simulink model "Fusion_Frame_Model_Architecture"  (R2018a)
settings: Solver=FixedStepAuto  StartTime=0.0  StopTime=SimulationTime  FixedStep=SamplingTime  RelTol=1e-3
undefined symbols (not defined in the file or in its folder): ACTIVATE_CAM, ACTIVATE_RAD, CAM1_detTimeStamp, CAM1_MeasNoise, CAM1_objClassID, CAM1_PX, CAM1_PY, CAM1_VX, CAM1_VY, CAM2_detTimeStamp, CAM2_MeasNoise, CAM2_objClassID, CAM2_PX, CAM2_PY, CAM2_VX, CAM2_VY, CAM3_detTimeStamp, CAM3_MeasNoise, CAM3_objClassID, CAM3_PX, CAM3_PY, CAM3_VX, CAM3_VY, CAM4_detTimeStamp, CAM4_MeasNoise, CAM4_objClassID, CAM4_PX, CAM4_PY, CAM4_VX, CAM4_VY, CAM5_detTimeStamp, CAM5_MeasNoise, CAM5_objClassID, CAM5_PX, CAM5_PY, CAM5_VX, CAM5_VY, CAM6_detTimeStamp, CAM6_MeasNoise, CAM6_objClassID, CAM6_PX, CAM6_PY, CAM6_VX, CAM6_VY, CAM7_detTimeStamp, CAM7_MeasNoise, CAM7_objClassID, CAM7_PX, CAM7_PY, CAM7_VX, CAM7_VY, CAM8_detTimeStamp, CAM8_MeasNoise, CAM8_objClassID, CAM8_PX, CAM8_PY, CAM8_VX, CAM8_VY, CAM_nMeas, CAM_TYPE ... (+181)
libraries: simulink_extras x4
(part 7 of 11)

== system Fusion_Frame_Model_Architecture/SENSOR_MEASUREMENTS/RADAR_CAMERA_EGO_SENSOR_INTERFACE/RoadSensors/Camera6/ExtractMeasParam1 ==
  idx : Inport
  time : Inport  Port=2
  Constant : Constant  Value=LINE_CURVATURE_CAM6
  Constant1 : Constant  Value=LINE_CURVDERIVATIVE_CAM6
  Constant2 : Constant  Value=LINE_CURVELENGTH_CAM6
  Constant3 : Constant  Value=LINE_HEADINGANGLE_CAM6
  Constant4 : Constant  Value=LINE_LATERALOFFSET_CAM6
  Constant5 : Constant  Value=LINE_XMIN_CAM6
  Constant6 : Constant  Value=LINE_detTimeStamp_CAM6
  Constant7 : Constant  Value=LINE_XMAX_CAM6
  Constant8 : Constant  Value=LINE_WIDTH_CAM6
  CurvLength : Selector  NumberOfDimensions=2  InputPortWidth=3  IndexOptions=Index vector (port),Index vector (port)  Indices=[1 3],1  OutputSizes=1,1
  Curvature : Selector  NumberOfDimensions=2  InputPortWidth=3  IndexOptions=Index vector (port),Index vector (port)  Indices=[1 3],1  OutputSizes=1,1
  CurvatureRate : Selector  NumberOfDimensions=2  InputPortWidth=3  IndexOptions=Index vector (port),Index vector (port)  Indices=[1 3],1  OutputSizes=1,1
  HeadingAngle : Selector  NumberOfDimensions=2  InputPortWidth=3  IndexOptions=Index vector (port),Index vector (port)  Indices=[1 3],1  OutputSizes=1,1
  LateralOffset : Selector  NumberOfDimensions=2  InputPortWidth=3  IndexOptions=Index vector (port),Index vector (port)  Indices=[1 3],1  OutputSizes=1,1
  lineWidth : Selector  NumberOfDimensions=2  InputPortWidth=3  IndexOptions=Index vector (port),Index vector (port)  Indices=[1 3],1  OutputSizes=1,1
  minValidX : Selector  NumberOfDimensions=2  InputPortWidth=3  IndexOptions=Index vector (port),Index vector (port)  Indices=[1 3],1  OutputSizes=1,1
  minValidY : Selector  NumberOfDimensions=2  InputPortWidth=3  IndexOptions=Index vector (port),Index vector (port)  Indices=[1 3],1  OutputSizes=1,1
  timeStamp : Selector  NumberOfDimensions=2  InputPortWidth=3  IndexOptions=Select all,Index vector (port)  Indices=[1 3],1  OutputSizes=1,1
  curvature : Outport
  curvRate : Outport  Port=2
  curvLength : Outport  Port=3
  headingAngle : Outport  Port=4
  lateralOffset : Outport  Port=5
  xmin : Outport  Port=6
  xmax : Outport  Port=7
  lineMarkWidth : Outport  Port=8
  measCaptureTime : Outport  Port=9
  wires:
  Constant3/1 -> HeadingAngle/1
  Constant2/1 -> CurvLength/1
  HeadingAngle/1 -> headingAngle/1
  Constant/1 -> Curvature/1
  Constant1/1 -> CurvatureRate/1
  CurvLength/1 -> curvLength/1
  Curvature/1 -> curvature/1
  CurvatureRate/1 -> curvRate/1
  Constant4/1 -> LateralOffset/1
  Constant5/1 -> minValidX/1
  Constant6/1 -> timeStamp/1
  timeStamp/1 -> measCaptureTime/1
  minValidX/1 -> xmin/1
  LateralOffset/1 -> lateralOffset/1
  minValidY/1 -> xmax/1
  Constant7/1 -> minValidY/1
  lineWidth/1 -> lineMarkWidth/1
  time/1 -> minValidX/2, minValidY/2, lineWidth/2, timeStamp/2, LateralOffset/2, HeadingAngle/2, CurvLength/2, CurvatureRate/2, Curvature/2
  idx/1 -> minValidX/3, lineWidth/3, minValidY/3, LateralOffset/3, HeadingAngle/3, CurvLength/3, CurvatureRate/3, Curvature/3
  Constant8/1 -> lineWidth/1

== system Fusion_Frame_Model_Architecture/SENSOR_MEASUREMENTS/RADAR_CAMERA_EGO_SENSOR_INTERFACE/RoadSensors/Camera6/IsValid2 ==
  LineID : Inport
  curvature : Inport  Port=2
  curvatureRate : Inport  Port=3
  curvLength : Inport  Port=4
  HeadingAngle : Inport  Port=5
  Abs{,1..3} (4 alike) : Abs
  Add : Sum  Inputs=++++
  Constant : Constant  Value=uint16(0)
  Data Type Conversion : DataTypeConversion  OutDataTypeStr=uint16
  Switch : Switch  Threshold=0.000001
  validID : Outport
  wires:
  Add/1 -> Switch/2
  Abs2/1 -> Add/3
  Constant/1 -> Switch/3
  Abs/1 -> Add/1
  curvature/1 -> Abs/1
  Abs3/1 -> Add/4
  Abs1/1 -> Add/2
  HeadingAngle/1 -> Abs3/1
  curvatureRate/1 -> Abs1/1
  curvLength/1 -> Abs2/1
  LineID/1 -> Data Type Conversion/1
  Switch/1 -> validID/1
  Data Type Conversion/1 -> Switch/1

== system Fusion_Frame_Model_Architecture/SENSOR_MEASUREMENTS/RADAR_CAMERA_EGO_SENSOR_INTERFACE/RoadSensors/Camera6/Subsystem1 ==
  CameraLineCoeff : Inport
  curv : Inport  Port=2
  curvRate : Inport  Port=3
  curvLen : Inport  Port=4
  alpha : Inport  Port=5
  ValidID : Inport  Port=6
  lateralOffset : Inport  Port=7
  xmin : Inport  Port=8
  xmax : Inport  Port=9
  lineWidth : Inport  Port=10
  TIME_STAMP : Inport  Port=11
  iter : Inport  Port=12
  Assignment : Assignment  DiagnosticForDimensions=Warning  IndexOptions=Index vector (port)  Indices=1  OutputSizes=1
  Bus Creator1 : BusCreator  Inputs=11  OutDataTypeStr=Bus: LineMeasParam  NonVirtualBus=on
  Bus Creator2 : BusCreator  Inputs=11  OutDataTypeStr=Bus: LineMeasParam  NonVirtualBus=on
  Constant1 : Constant  Value=single(10)
  Constant14 : Constant  Value=uint8(6)
  Constant2 : Constant  Value=single(10)
  Constant{35..39,43} (6 alike) : Constant  Value=single(0)
  Constant44 : Constant  Value=single(10)
  Switch : Switch  Criteria=u2 ~= 0
  C1 : Outport
  wires:
  Bus Creator1/1 -> Switch/3
  ValidID/1 -> Bus Creator1/2, Switch/2, Bus Creator2/2  "lineID"
  Bus Creator2/1 -> Switch/1
  CameraLineCoeff/1 -> Assignment/1
  Switch/1 -> Assignment/2
  iter/1 -> Assignment/3
  Assignment/1 -> C1/1
  TIME_STAMP/1 -> Bus Creator2/1  "TimeStamp"
  curv/1 -> Bus Creator2/4  "curvature"
  curvRate/1 -> Bus Creator2/5  "curvatureRate"
  curvLen/1 -> Bus Creator2/6  "curveLength"
  alpha/1 -> Bus Creator2/7  "HeadingAngle"
  lateralOffset/1 -> Bus Creator2/8  "LateralOffset"
  lineWidth/1 -> Bus Creator2/11  "LineMarkWidth"
  xmax/1 -> Bus Creator2/10  "validMinLongCoordLine"
  xmin/1 -> Bus Creator2/9  "validMaxLongCoordLine"
  Constant35/1 -> Bus Creator1/1  "TimeStamp"
  Constant14/1 -> Bus Creator2/3, Bus Creator1/3  "cameraID"
  Constant36/1 -> Bus Creator1/4  "curvature"
  Constant37/1 -> Bus Creator1/5  "curvatureRate"
  Constant38/1 -> Bus Creator1/6  "curveLength"
  Constant39/1 -> Bus Creator1/7  "HeadingAngle"
  Constant43/1 -> Bus Creator1/8  "LateralOffset"
  Constant44/1 -> Bus Creator1/9  "validMaxLongCoordLine"
  Constant1/1 -> Bus Creator1/10  "validMinLongCoordLine"
  Constant2/1 -> Bus Creator1/11  "LineMarkWidth"

== system Fusion_Frame_Model_Architecture/SENSOR_MEASUREMENTS/RADAR_CAMERA_EGO_SENSOR_INTERFACE/RoadSensors/Camera7/ExtractMeasParam1 ==
  idx : Inport
  time : Inport  Port=2
  Constant : Constant  Value=LINE_CURVATURE_CAM7
  Constant1 : Constant  Value=LINE_CURVDERIVATIVE_CAM7
  Constant2 : Constant  Value=LINE_CURVELENGTH_CAM7
  Constant3 : Constant  Value=LINE_HEADINGANGLE_CAM7
  Constant4 : Constant  Value=LINE_LATERALOFFSET_CAM7
  Constant5 : Constant  Value=LINE_XMIN_CAM7
  Constant6 : Constant  Value=LINE_detTimeStamp_CAM7
  Constant7 : Constant  Value=LINE_XMAX_CAM7
  Constant8 : Constant  Value=LINE_WIDTH_CAM7
  CurvLength : Selector  NumberOfDimensions=2  InputPortWidth=3  IndexOptions=Index vector (port),Index vector (port)  Indices=[1 3],1  OutputSizes=1,1
  Curvature : Selector  NumberOfDimensions=2  InputPortWidth=3  IndexOptions=Index vector (port),Index vector (port)  Indices=[1 3],1  OutputSizes=1,1
  CurvatureRate : Selector  NumberOfDimensions=2  InputPortWidth=3  IndexOptions=Index vector (port),Index vector (port)  Indices=[1 3],1  OutputSizes=1,1
  HeadingAngle : Selector  NumberOfDimensions=2  InputPortWidth=3  IndexOptions=Index vector (port),Index vector (port)  Indices=[1 3],1  OutputSizes=1,1
  LateralOffset : Selector  NumberOfDimensions=2  InputPortWidth=3  IndexOptions=Index vector (port),Index vector (port)  Indices=[1 3],1  OutputSizes=1,1
  lineWidth : Selector  NumberOfDimensions=2  InputPortWidth=3  IndexOptions=Index vector (port),Index vector (port)  Indices=[1 3],1  OutputSizes=1,1
  minValidX : Selector  NumberOfDimensions=2  InputPortWidth=3  IndexOptions=Index vector (port),Index vector (port)  Indices=[1 3],1  OutputSizes=1,1
  minValidY : Selector  NumberOfDimensions=2  InputPortWidth=3  IndexOptions=Index vector (port),Index vector (port)  Indices=[1 3],1  OutputSizes=1,1
  timeStamp : Selector  NumberOfDimensions=2  InputPortWidth=3  IndexOptions=Select all,Index vector (port)  Indices=[1 3],1  OutputSizes=1,1
  curvature : Outport
  curvRate : Outport  Port=2
  curvLength : Outport  Port=3
  headingAngle : Outport  Port=4
  lateralOffset : Outport  Port=5
  xmin : Outport  Port=6
  xmax : Outport  Port=7
  lineMarkWidth : Outport  Port=8
  measCaptureTime : Outport  Port=9
  wires:
  Constant3/1 -> HeadingAngle/1
  Constant2/1 -> CurvLength/1
  HeadingAngle/1 -> headingAngle/1
  Constant/1 -> Curvature/1
  Constant1/1 -> CurvatureRate/1
  CurvLength/1 -> curvLength/1
  Curvature/1 -> curvature/1
  CurvatureRate/1 -> curvRate/1
  Constant4/1 -> LateralOffset/1
  Constant5/1 -> minValidX/1
  Constant6/1 -> timeStamp/1
  timeStamp/1 -> measCaptureTime/1
  minValidX/1 -> xmin/1
  LateralOffset/1 -> lateralOffset/1
  minValidY/1 -> xmax/1
  Constant7/1 -> minValidY/1
  lineWidth/1 -> lineMarkWidth/1
  time/1 -> minValidX/2, minValidY/2, lineWidth/2, timeStamp/2, LateralOffset/2, HeadingAngle/2, CurvLength/2, CurvatureRate/2, Curvature/2
  idx/1 -> minValidX/3, lineWidth/3, minValidY/3, LateralOffset/3, HeadingAngle/3, CurvLength/3, CurvatureRate/3, Curvature/3
  Constant8/1 -> lineWidth/1

== system Fusion_Frame_Model_Architecture/SENSOR_MEASUREMENTS/RADAR_CAMERA_EGO_SENSOR_INTERFACE/RoadSensors/Camera7/IsValid2 ==
  LineID : Inport
  curvature : Inport  Port=2
  curvatureRate : Inport  Port=3
  curvLength : Inport  Port=4
  HeadingAngle : Inport  Port=5
  Abs{,1..3} (4 alike) : Abs
  Add : Sum  Inputs=++++
  Constant : Constant  Value=uint16(0)
  Data Type Conversion : DataTypeConversion  OutDataTypeStr=uint16
  Switch : Switch  Threshold=0.000001
  validID : Outport
  wires:
  Add/1 -> Switch/2
  Abs2/1 -> Add/3
  Constant/1 -> Switch/3
  Abs/1 -> Add/1
  curvature/1 -> Abs/1
  Abs3/1 -> Add/4
  Abs1/1 -> Add/2
  HeadingAngle/1 -> Abs3/1
  curvatureRate/1 -> Abs1/1
  curvLength/1 -> Abs2/1
  LineID/1 -> Data Type Conversion/1
  Switch/1 -> validID/1
  Data Type Conversion/1 -> Switch/1

== system Fusion_Frame_Model_Architecture/SENSOR_MEASUREMENTS/RADAR_CAMERA_EGO_SENSOR_INTERFACE/RoadSensors/Camera7/Subsystem1 ==
  CameraLineCoeff : Inport
  curv : Inport  Port=2
  curvRate : Inport  Port=3
  curvLen : Inport  Port=4
  alpha : Inport  Port=5
  ValidID : Inport  Port=6
  lateralOffset : Inport  Port=7
  xmin : Inport  Port=8
  xmax : Inport  Port=9
  lineWidth : Inport  Port=10
  TIME_STAMP : Inport  Port=11
  iter : Inport  Port=12
  Assignment : Assignment  DiagnosticForDimensions=Warning  IndexOptions=Index vector (port)  Indices=1  OutputSizes=1
  Bus Creator1 : BusCreator  Inputs=11  OutDataTypeStr=Bus: LineMeasParam  NonVirtualBus=on
  Bus Creator2 : BusCreator  Inputs=11  OutDataTypeStr=Bus: LineMeasParam  NonVirtualBus=on
  Constant1 : Constant  Value=single(10)
  Constant14 : Constant  Value=uint8(7)
  Constant2 : Constant  Value=single(10)
  Constant{35..39,43} (6 alike) : Constant  Value=single(0)
  Constant44 : Constant  Value=single(10)
  Switch : Switch  Criteria=u2 ~= 0
  C1 : Outport
  wires:
  Bus Creator1/1 -> Switch/3
  ValidID/1 -> Bus Creator1/2, Switch/2, Bus Creator2/2  "lineID"
  Bus Creator2/1 -> Switch/1
  CameraLineCoeff/1 -> Assignment/1
  Switch/1 -> Assignment/2
  iter/1 -> Assignment/3
  Assignment/1 -> C1/1
  TIME_STAMP/1 -> Bus Creator2/1  "TimeStamp"
  curv/1 -> Bus Creator2/4  "curvature"
  curvRate/1 -> Bus Creator2/5  "curvatureRate"
  curvLen/1 -> Bus Creator2/6  "curveLength"
  alpha/1 -> Bus Creator2/7  "HeadingAngle"
  lateralOffset/1 -> Bus Creator2/8  "LateralOffset"
  lineWidth/1 -> Bus Creator2/11  "LineMarkWidth"
  xmax/1 -> Bus Creator2/10  "validMinLongCoordLine"
  xmin/1 -> Bus Creator2/9  "validMaxLongCoordLine"
  Constant35/1 -> Bus Creator1/1  "TimeStamp"
  Constant14/1 -> Bus Creator2/3, Bus Creator1/3  "cameraID"
  Constant36/1 -> Bus Creator1/4  "curvature"
  Constant37/1 -> Bus Creator1/5  "curvatureRate"
  Constant38/1 -> Bus Creator1/6  "curveLength"
  Constant39/1 -> Bus Creator1/7  "HeadingAngle"
  Constant43/1 -> Bus Creator1/8  "LateralOffset"
  Constant44/1 -> Bus Creator1/9  "validMaxLongCoordLine"
  Constant1/1 -> Bus Creator1/10  "validMinLongCoordLine"
  Constant2/1 -> Bus Creator1/11  "LineMarkWidth"

== system Fusion_Frame_Model_Architecture/SENSOR_MEASUREMENTS/RADAR_CAMERA_EGO_SENSOR_INTERFACE/RoadSensors/Camera8/ExtractMeasParam1 ==
  idx : Inport
  time : Inport  Port=2
  Constant : Constant  Value=LINE_CURVATURE_CAM8
  Constant1 : Constant  Value=LINE_CURVDERIVATIVE_CAM8
  Constant2 : Constant  Value=LINE_CURVELENGTH_CAM8
  Constant3 : Constant  Value=LINE_HEADINGANGLE_CAM8
  Constant4 : Constant  Value=LINE_LATERALOFFSET_CAM8
  Constant5 : Constant  Value=LINE_XMIN_CAM8
  Constant6 : Constant  Value=LINE_detTimeStamp_CAM8
  Constant7 : Constant  Value=LINE_XMAX_CAM8
  Constant8 : Constant  Value=LINE_WIDTH_CAM8
  CurvLength : Selector  NumberOfDimensions=2  InputPortWidth=3  IndexOptions=Index vector (port),Index vector (port)  Indices=[1 3],1  OutputSizes=1,1
  Curvature : Selector  NumberOfDimensions=2  InputPortWidth=3  IndexOptions=Index vector (port),Index vector (port)  Indices=[1 3],1  OutputSizes=1,1
  CurvatureRate : Selector  NumberOfDimensions=2  InputPortWidth=3  IndexOptions=Index vector (port),Index vector (port)  Indices=[1 3],1  OutputSizes=1,1
  HeadingAngle : Selector  NumberOfDimensions=2  InputPortWidth=3  IndexOptions=Index vector (port),Index vector (port)  Indices=[1 3],1  OutputSizes=1,1
  LateralOffset : Selector  NumberOfDimensions=2  InputPortWidth=3  IndexOptions=Index vector (port),Index vector (port)  Indices=[1 3],1  OutputSizes=1,1
  lineWidth : Selector  NumberOfDimensions=2  InputPortWidth=3  IndexOptions=Index vector (port),Index vector (port)  Indices=[1 3],1  OutputSizes=1,1
  minValidX : Selector  NumberOfDimensions=2  InputPortWidth=3  IndexOptions=Index vector (port),Index vector (port)  Indices=[1 3],1  OutputSizes=1,1
  minValidY : Selector  NumberOfDimensions=2  InputPortWidth=3  IndexOptions=Index vector (port),Index vector (port)  Indices=[1 3],1  OutputSizes=1,1
  timeStamp : Selector  NumberOfDimensions=2  InputPortWidth=3  IndexOptions=Select all,Index vector (port)  Indices=[1 3],1  OutputSizes=1,1
  curvature : Outport
  curvRate : Outport  Port=2
  curvLength : Outport  Port=3
  headingAngle : Outport  Port=4
  lateralOffset : Outport  Port=5
  xmin : Outport  Port=6
  xmax : Outport  Port=7
  lineMarkWidth : Outport  Port=8
  measCaptureTime : Outport  Port=9
  wires:
  Constant3/1 -> HeadingAngle/1
  Constant2/1 -> CurvLength/1
  HeadingAngle/1 -> headingAngle/1
  Constant/1 -> Curvature/1
  Constant1/1 -> CurvatureRate/1
  CurvLength/1 -> curvLength/1
  Curvature/1 -> curvature/1
  CurvatureRate/1 -> curvRate/1
  Constant4/1 -> LateralOffset/1
  Constant5/1 -> minValidX/1
  Constant6/1 -> timeStamp/1
  timeStamp/1 -> measCaptureTime/1
  minValidX/1 -> xmin/1
  LateralOffset/1 -> lateralOffset/1
  minValidY/1 -> xmax/1
  Constant7/1 -> minValidY/1
  lineWidth/1 -> lineMarkWidth/1
  time/1 -> minValidX/2, minValidY/2, lineWidth/2, timeStamp/2, LateralOffset/2, HeadingAngle/2, CurvLength/2, CurvatureRate/2, Curvature/2
  idx/1 -> minValidX/3, lineWidth/3, minValidY/3, LateralOffset/3, HeadingAngle/3, CurvLength/3, CurvatureRate/3, Curvature/3
  Constant8/1 -> lineWidth/1

== system Fusion_Frame_Model_Architecture/SENSOR_MEASUREMENTS/RADAR_CAMERA_EGO_SENSOR_INTERFACE/RoadSensors/Camera8/IsValid2 ==
  LineID : Inport
  curvature : Inport  Port=2
  curvatureRate : Inport  Port=3
  curvLength : Inport  Port=4
  HeadingAngle : Inport  Port=5
  Abs{,1..3} (4 alike) : Abs
  Add : Sum  Inputs=++++
  Constant : Constant  Value=uint16(0)
  Data Type Conversion : DataTypeConversion  OutDataTypeStr=uint16
  Switch : Switch  Threshold=0.000001
  validID : Outport
  wires:
  Add/1 -> Switch/2
  Abs2/1 -> Add/3
  Constant/1 -> Switch/3
  Abs/1 -> Add/1
  curvature/1 -> Abs/1
  Abs3/1 -> Add/4
  Abs1/1 -> Add/2
  HeadingAngle/1 -> Abs3/1
  curvatureRate/1 -> Abs1/1
  curvLength/1 -> Abs2/1
  LineID/1 -> Data Type Conversion/1
  Switch/1 -> validID/1
  Data Type Conversion/1 -> Switch/1

== system Fusion_Frame_Model_Architecture/SENSOR_MEASUREMENTS/RADAR_CAMERA_EGO_SENSOR_INTERFACE/RoadSensors/Camera8/Subsystem1 ==
  CameraLineCoeff : Inport
  curv : Inport  Port=2
  curvRate : Inport  Port=3
  curvLen : Inport  Port=4
  alpha : Inport  Port=5
  ValidID : Inport  Port=6
  lateralOffset : Inport  Port=7
  xmin : Inport  Port=8
  xmax : Inport  Port=9
  lineWidth : Inport  Port=10
  TIME_STAMP : Inport  Port=11
  iter : Inport  Port=12
  Assignment : Assignment  DiagnosticForDimensions=Warning  IndexOptions=Index vector (port)  Indices=1  OutputSizes=1
  Bus Creator1 : BusCreator  Inputs=11  OutDataTypeStr=Bus: LineMeasParam  NonVirtualBus=on
  Bus Creator2 : BusCreator  Inputs=11  OutDataTypeStr=Bus: LineMeasParam  NonVirtualBus=on
  Constant1 : Constant  Value=single(10)
  Constant14 : Constant  Value=uint8(8)
  Constant2 : Constant  Value=single(10)
  Constant{35..39,43} (6 alike) : Constant  Value=single(0)
  Constant44 : Constant  Value=single(10)
  Switch : Switch  Criteria=u2 ~= 0
  C1 : Outport
  wires:
  Bus Creator1/1 -> Switch/3
  ValidID/1 -> Bus Creator1/2, Switch/2, Bus Creator2/2  "lineID"
  Bus Creator2/1 -> Switch/1
  CameraLineCoeff/1 -> Assignment/1
  Switch/1 -> Assignment/2
  iter/1 -> Assignment/3
  Assignment/1 -> C1/1
  TIME_STAMP/1 -> Bus Creator2/1  "TimeStamp"
  curv/1 -> Bus Creator2/4  "curvature"
  curvRate/1 -> Bus Creator2/5  "curvatureRate"
  curvLen/1 -> Bus Creator2/6  "curveLength"
  alpha/1 -> Bus Creator2/7  "HeadingAngle"
  lateralOffset/1 -> Bus Creator2/8  "LateralOffset"
  lineWidth/1 -> Bus Creator2/11  "LineMarkWidth"
  xmax/1 -> Bus Creator2/10  "validMinLongCoordLine"
  xmin/1 -> Bus Creator2/9  "validMaxLongCoordLine"
  Constant35/1 -> Bus Creator1/1  "TimeStamp"
  Constant14/1 -> Bus Creator2/3, Bus Creator1/3  "cameraID"
  Constant36/1 -> Bus Creator1/4  "curvature"
  Constant37/1 -> Bus Creator1/5  "curvatureRate"
  Constant38/1 -> Bus Creator1/6  "curveLength"
  Constant39/1 -> Bus Creator1/7  "HeadingAngle"
  Constant43/1 -> Bus Creator1/8  "LateralOffset"
  Constant44/1 -> Bus Creator1/9  "validMaxLongCoordLine"
  Constant1/1 -> Bus Creator1/10  "validMinLongCoordLine"
  Constant2/1 -> Bus Creator1/11  "LineMarkWidth"

== system Fusion_Frame_Model_Architecture/SENSOR_FUSION_SYSTEM/OBJECT_TRACKER_SENSOR_FUSION/CAMERA_HOMOGENEOUS_FUSION/GATING/MEASUREMENT_TO_TRACK_GATING_AND_LOGLIKELIHOOD_COMPUTATION/GATE_MEASUREMENTS_AND_COMPUTE_LIKELIHOOD ==
  GatedMeasFlagArrayIn : Inport
  Meas : Inport  Port=2
  nMeas : Inport  Port=3
  TrackStateVector : Inport  Port=4
  TrackErrCov : Inport  Port=5
  TrackIdx : Inport  Port=6
  LogLikelihoodArrayIn : Inport  Port=7
  For Iterator : ForIterator  ResetStates=reset  IterationSource=external
  Terminator{,1..4} (5 alike) : Terminator
  GatedMeasFlagArray : Outport
  LogLikelihoodArray : Outport  Port=2
  wires:
  nMeas/1 -> For Iterator/1
  Meas/1 -> Terminator3/1
  TrackErrCov/1 -> Terminator1/1
  TrackStateVector/1 -> Terminator2/1
  GatedMeasFlagArrayIn/1 -> GatedMeasFlagArray/1
  LogLikelihoodArrayIn/1 -> LogLikelihoodArray/1
  TrackIdx/1 -> Terminator/1
  For Iterator/1 -> Terminator4/1

== system Fusion_Frame_Model_Architecture/SENSOR_FUSION_SYSTEM/OBJECT_TRACKER_SENSOR_FUSION/CAMERA_HOMOGENEOUS_FUSION/GATING/MEASUREMENT_TO_TRACK_GATING_AND_LOGLIKELIHOOD_COMPUTATION/GET_DATA ==
  Meas : Inport
  TrackParamPred : Inport  Port=2
  TrackIdx : Inport  Port=3
  Bus Selector : BusSelector  OutputSignals=StateParam
  Bus Selector1 : BusSelector  OutputSignals=px,vx,ax,py,vy,ay,ErrCOV
  Bus Selector2 : BusSelector  OutputSignals=ValidCumulativeMeasCount
  Mux : Mux  Inputs=6
  Reshape : Reshape  OutputDimensionality=Column vector (2-D)
  Selector : Selector  InputPortWidth=100  IndexOptions=Index vector (port)  Indices=[1 3]  OutputSizes=1
  Selector1 : Selector  NumberOfDimensions=2  InputPortWidth=3  IndexOptions=Select all,Index vector (port)  Indices=[1 3],1  OutputSizes=1,1
  Width : Width
  nMeas : Outport
  StateVector : Outport  Port=2
  StateErrCov : Outport  Port=3
  wires:
  TrackParamPred/1 -> Selector/1
  TrackIdx/1 -> Selector/2
  Selector/1 -> Bus Selector/1
  Reshape/1 -> StateVector/1
  Bus Selector/1 -> Bus Selector1/1  "<StateParam>"
  Bus Selector1/7 -> StateErrCov/1  "<ErrCOV>"
  Bus Selector1/1 -> Mux/1  "<px>"
  Bus Selector1/2 -> Mux/2  "<vx>"
  Bus Selector1/3 -> Mux/3  "<ax>"
  Bus Selector1/4 -> Mux/4  "<py>"
  Bus Selector1/5 -> Mux/5  "<vy>"
  Bus Selector1/6 -> Mux/6  "<ay>"
  Mux/1 -> Reshape/1
  Meas/1 -> Bus Selector2/1
  Bus Selector2/1 -> Width/1, Selector1/1  "<ValidCumulativeMeasCount>"
  Width/1 -> Selector1/2
  Selector1/1 -> nMeas/1

== system Fusion_Frame_Model_Architecture/SENSOR_FUSION_SYSTEM/OBJECT_TRACKER_SENSOR_FUSION/CAMERA_HOMOGENEOUS_FUSION/NEAREST_NEIGHBOUR_CLUSTERING_FOR_CAMERA_MEASUREMENT/NN_MEASUREMENT_GROUPING_WITHIN_EPS/COMPUTE_MEAN_IF_CLUSTER_FORMED ==
  meas : Inport
  CLSTR_DATA : Inport  Port=2
  Enable : EnablePort
  COMPUTE_COVARIANCE : Subsystem
  COMPUTE_COVARIANCE_SUM : Subsystem  TreatAsAtomicUnit=on
  COMPUTE_MEAN : Subsystem
  COMPUTE_MEAN_SUM : Subsystem  TreatAsAtomicUnit=on
  GET_DATA : Subsystem
  CLSTR_CNTR_UPD : Outport
  CLSTR_COV_UPD : Outport  Port=2
  wires:
  GET_DATA/1(nPts) -> [nPts], COMPUTE_MEAN_SUM/2(nPoints), COMPUTE_MEAN/2(n), COMPUTE_COVARIANCE_SUM/3(nPoints)
  GET_DATA/2(<ClusterMember>) -> COMPUTE_COVARIANCE_SUM/4(ClusterMembers), [ClstrMembers]
  [Meas] -> COMPUTE_COVARIANCE_SUM/2(MeasArray)
  meas/1 -> [Meas], COMPUTE_MEAN_SUM/3(MeasArray)
  [ClstrMembers] -> COMPUTE_MEAN_SUM/1(ClusterMembers)
  COMPUTE_COVARIANCE/1(Covariance) -> CLSTR_COV_UPD/1
  [nPts] -> COMPUTE_COVARIANCE/2(n)
  COMPUTE_MEAN/1(mean) -> CLSTR_CNTR_UPD/1, COMPUTE_COVARIANCE_SUM/1(mean)
  CLSTR_DATA/1 -> GET_DATA/1(CLSTR)
  COMPUTE_MEAN_SUM/1(ClusterMeanSUM) -> COMPUTE_MEAN/1(mean_sum)
  COMPUTE_COVARIANCE_SUM/1(ClusterCovSUM) -> COMPUTE_COVARIANCE/1(covariance_sum)

== system Fusion_Frame_Model_Architecture/SENSOR_FUSION_SYSTEM/OBJECT_TRACKER_SENSOR_FUSION/CAMERA_HOMOGENEOUS_FUSION/NEAREST_NEIGHBOUR_CLUSTERING_FOR_CAMERA_MEASUREMENT/NN_MEASUREMENT_GROUPING_WITHIN_EPS/For Iterator Subsystem ==
  idx_i : Inport
  measArray : Inport  Port=2
  CLSTR_DATA : Inport  Port=3
  If : If  IfExpression=u1 ~= 0
  If Action Subsystem : Subsystem  TreatAsAtomicUnit=on
  MERGE_SIGNALS : Subsystem
  NN : Subsystem
  Subsystem : Subsystem
  nPts : Outport
  CLSTR_DATA_out : Outport  Port=2
  wires:
  idx_i/1 -> Subsystem/1(idx_i), NN/3(idx_i)
  CLSTR_DATA/1 -> Subsystem/2(CLSTR_in)
  Subsystem/1(isNotVisited) -> If/1
  If/1 -> NN/Action
  If/2 -> If Action Subsystem/Action
  measArray/1 -> NN/2(measArray)
  If Action Subsystem/1(CLSTR_DATA_NO_UPD) -> MERGE_SIGNALS/1(CLSTR_NO_UPD)
  If Action Subsystem/2(nPtsEpsNoUpd) -> MERGE_SIGNALS/2(nPtsEpsNoUpd)
  NN/1(nPtsEps) -> MERGE_SIGNALS/3(nPtsUpd)
  MERGE_SIGNALS/2(CLSTR_DATA) -> CLSTR_DATA_out/1
  Subsystem/2(CLSTR_out) -> NN/1(CLSTR_DATA), If Action Subsystem/1(CLSTR_DATA)
  NN/2(CLSTR_DATA_UPD) -> MERGE_SIGNALS/4(CLSTR_UPD)
  MERGE_SIGNALS/1(nPtsEps) -> nPts/1

== system Fusion_Frame_Model_Architecture/SENSOR_FUSION_SYSTEM/OBJECT_TRACKER_SENSOR_FUSION/CAMERA_HOMOGENEOUS_FUSION/NEAREST_NEIGHBOUR_CLUSTERING_FOR_CAMERA_MEASUREMENT/NN_MEASUREMENT_GROUPING_WITHIN_EPS/Subsystem1 ==
  CLSTR_DATA : Inport
  Constant : Constant  Value=uint16(0)
  GreaterThan : RelationalOperator  Operator=>  OutDataTypeStr=boolean  RndMeth=Simplest
  Logical Operator : Logic  Operator=NOT  AllPortsSameDT=off  OutDataTypeStr=boolean
  NoUpd : Outport
  Upd : Outport  Port=2
  wires:
  CLSTR_DATA/1 -> GreaterThan/1
  GreaterThan/1 -> Logical Operator/1, Upd/1
  Constant/1 -> GreaterThan/2
  Logical Operator/1 -> NoUpd/1

== system Fusion_Frame_Model_Architecture/SENSOR_FUSION_SYSTEM/OBJECT_TRACKER_SENSOR_FUSION/CAMERA_HOMOGENEOUS_FUSION/NEAREST_NEIGHBOUR_CLUSTERING_FOR_CAMERA_MEASUREMENT/NN_MEASUREMENT_GROUPING_WITHIN_EPS/Subsystem2 ==
  Enable : EnablePort
  Constant : Constant  Value=single(zeros(2,1))  VectorParams1D=off
  Constant1 : Constant  Value=single(zeros(2,2))  VectorParams1D=off
  Mean : Outport
  Cov : Outport  Port=2
  wires:
  Constant/1 -> Mean/1
  Constant1/1 -> Cov/1

== system Fusion_Frame_Model_Architecture/SENSOR_FUSION_SYSTEM/OBJECT_TRACKER_SENSOR_FUSION/CAMERA_HOMOGENEOUS_FUSION/NEAREST_NEIGHBOUR_CLUSTERING_FOR_CAMERA_MEASUREMENT/NN_MEASUREMENT_GROUPING_WITHIN_EPS/Subsystem3 ==
  MeanNoUpd : Inport
  CovNoUpd : Inport  Port=2
  MeanUpd : Inport  Port=3
  CovUpd : Inport  Port=4
  CLSTR_DATA : Inport  Port=5
  Flag : Inport  Port=6
  GET_DATA_FROM_BUS : Subsystem
  SET_DATA_TO_BUS : Subsystem
  UPDATE_CLUSTER_DATA : Subsystem
  CLSTR_DATA_UPD : Outport
  wires:
  GET_DATA_FROM_BUS/1(<ClusterCenter>) -> UPDATE_CLUSTER_DATA/1(Center_ARRAY)
  GET_DATA_FROM_BUS/2(<ClusterCovariance>) -> UPDATE_CLUSTER_DATA/2(Cov_ARRAY)
  GET_DATA_FROM_BUS/3(<nClusters>) -> UPDATE_CLUSTER_DATA/3(ID)
  UPDATE_CLUSTER_DATA/1(CenterUpd) -> SET_DATA_TO_BUS/2(Mean_ARRAY)
  UPDATE_CLUSTER_DATA/2(CovUpd) -> SET_DATA_TO_BUS/3(Cov_ARRAY)
  MeanUpd/1 -> UPDATE_CLUSTER_DATA/4(mean1)
  MeanNoUpd/1 -> UPDATE_CLUSTER_DATA/5(mean2)
  CovNoUpd/1 -> UPDATE_CLUSTER_DATA/7(Cov2)
  Flag/1 -> UPDATE_CLUSTER_DATA/8(FLAG)
  CovUpd/1 -> UPDATE_CLUSTER_DATA/6(Cov1)
  CLSTR_DATA/1 -> SET_DATA_TO_BUS/1(CLSTR_DATA), GET_DATA_FROM_BUS/1(CLSTR_DATA)
  SET_DATA_TO_BUS/1("CLSTR_DATA_UPD ") -> CLSTR_DATA_UPD/1

== system Fusion_Frame_Model_Architecture/SENSOR_FUSION_SYSTEM/OBJECT_TRACKER_SENSOR_FUSION/CAMERA_HOMOGENEOUS_FUSION/STATE_PREDICTION/TRACK_STATE_PREDICTION/GET_DATA ==
  TrackParamPred : Inport
  TrackIdx : Inport  Port=2
  Bus Selector : BusSelector  OutputSignals=StateParam
  Bus Selector1 : BusSelector  OutputSignals=px,vx,ax,py,vy,ay,ErrCOV
  Mux : Mux  Inputs=6
  Reshape : Reshape  OutputDimensionality=Column vector (2-D)
  Selector : Selector  NumberOfDimensions=2  InputPortWidth=100  IndexOptions=Select all,Index vector (port)  Indices=[1 3],1  OutputSizes=1,1
  StateVector : Outport
  StateErrCov : Outport  Port=2
  wires:
  TrackParamPred/1 -> Selector/1
  TrackIdx/1 -> Selector/2
  Selector/1 -> Bus Selector/1
  Reshape/1 -> StateVector/1
  Bus Selector/1 -> Bus Selector1/1  "<StateParam>"
  Bus Selector1/7 -> StateErrCov/1  "<ErrCOV>"
  Bus Selector1/1 -> Mux/1  "<px>"
  Bus Selector1/2 -> Mux/2  "<vx>"
  Bus Selector1/3 -> Mux/3  "<ax>"
  Bus Selector1/4 -> Mux/4  "<py>"
  Bus Selector1/5 -> Mux/5  "<vy>"
  Bus Selector1/6 -> Mux/6  "<ay>"
  Mux/1 -> Reshape/1

== system Fusion_Frame_Model_Architecture/SENSOR_FUSION_SYSTEM/OBJECT_TRACKER_SENSOR_FUSION/CAMERA_HOMOGENEOUS_FUSION/STATE_PREDICTION/TRACK_STATE_PREDICTION/SET_DATA ==
  StatePred : Inport
  PredStateErrCov : Inport  Port=2
  objIdx : Inport  Port=3
  StateParamArray : Inport  Port=4
  Assignment1 : Assignment  NumberOfDimensions=2  DiagnosticForDimensions=Warning  IndexOptions=Assign all,Index vector (port)  Indices=1,1  OutputSizes=1,1
  Bus Creator : BusCreator  Inputs=8  OutDataTypeStr=Bus: TrackParamBus  NonVirtualBus=on
      settings: InheritFromInputs=off
  Bus Creator1 : BusCreator  Inputs=7  OutDataTypeStr=Bus: StateParamBus  NonVirtualBus=on
      settings: InheritFromInputs=off
  Bus Selector : BusSelector  OutputSignals=id,StateParam,StateCamSpecificParam,StateRadSpecificParam,StateParamAccuracy,SensorCatch,TrackQuality,TrackStatus
  Selector : Selector  NumberOfDimensions=2  InputPortWidth=3  IndexOptions=Select all,Index vector (port)  Indices=[1 3],1  OutputSizes=1,1
  Selector1 : Selector  InputPortWidth=6  IndexOptions=Index vector (dialog)  Indices=1  OutputSizes=1
  Selector2 : Selector  InputPortWidth=6  IndexOptions=Index vector (dialog)  Indices=2  OutputSizes=1
  Selector3 : Selector  InputPortWidth=6  IndexOptions=Index vector (dialog)  Indices=3  OutputSizes=1
  Selector4 : Selector  InputPortWidth=6  IndexOptions=Index vector (dialog)  Indices=4  OutputSizes=1
  Selector5 : Selector  InputPortWidth=6  IndexOptions=Index vector (dialog)  Indices=5  OutputSizes=1
  Selector6 : Selector  InputPortWidth=6  IndexOptions=Index vector (dialog)  Indices=6  OutputSizes=1
  Terminator : Terminator
  StateParam : Outport
  wires:
  StatePred/1 -> Selector6/1, Selector5/1, Selector4/1, Selector1/1, Selector2/1, Selector3/1
  Selector2/1 -> Bus Creator1/2  "vx"
  Selector4/1 -> Bus Creator1/4  "py"
  Selector3/1 -> Bus Creator1/3  "ax"
  Selector5/1 -> Bus Creator1/5  "vy"
  Selector1/1 -> Bus Creator1/1  "px"
  Selector6/1 -> Bus Creator1/6  "ay"
  Bus Creator1/1 -> [idx]
  PredStateErrCov/1 -> Bus Creator1/7  "ErrCOV"
  Bus Selector/1 -> Bus Creator/1  "<id>"
  Bus Selector/3 -> Bus Creator/3  "<StateCamSpecificParam>"
  Bus Selector/4 -> Bus Creator/4  "<StateRadSpecificParam>"
  Bus Selector/5 -> Bus Creator/5  "<StateParamAccuracy>"
  Bus Selector/6 -> Bus Creator/6  "<SensorCatch>"
  Bus Selector/7 -> Bus Creator/7  "<TrackQuality>"
  Bus Selector/8 -> Bus Creator/8  "<TrackStatus>"
  StateParamArray/1 -> [TrackArray], Selector/1
  objIdx/1 -> [objIdx], Selector/2
  Selector/1 -> Bus Selector/1
  Bus Creator/1 -> Assignment1/2
  Assignment1/1 -> StateParam/1
  [objIdx] -> Assignment1/3
  [TrackArray] -> Assignment1/1
  Bus Selector/2 -> Terminator/1  "<StateParam>"
  [idx] -> Bus Creator/2

== system Fusion_Frame_Model_Architecture/SENSOR_FUSION_SYSTEM/OBJECT_TRACKER_SENSOR_FUSION/CAMERA_HOMOGENEOUS_FUSION/STATE_PREDICTION/TRACK_STATE_PREDICTION/StatePredictionLinearModels ==
  StateVectorCA : Inport
  PrevStateErrorCov : Inport  Port=2
  Add : Sum
  Constant : Constant  Value=StateTranMatrix_CA
  Constant1 : Constant  Value=ProcessNoiseCovMat_CA
  Matrix Multiply : Product  Multiplication=Matrix(*)
  Matrix Multiply1 : Product  Inputs=3  Multiplication=Matrix(*)
  Transpose : Math  Operator=transpose  SaturateOnIntegerOverflow=on
  StatePred : Outport
  PriorStateErrorCov : Outport  Port=2
  wires:
  Add/1 -> PriorStateErrorCov/1
  Matrix Multiply/1 -> StatePred/1
  StateVectorCA/1 -> Matrix Multiply/2
  Constant1/1 -> Add/2
  Transpose/1 -> Matrix Multiply1/3
  Matrix Multiply1/1 -> Add/1
  Constant/1 -> Transpose/1, Matrix Multiply1/1, Matrix Multiply/1
  PrevStateErrorCov/1 -> Matrix Multiply1/2

== system Fusion_Frame_Model_Architecture/SENSOR_FUSION_SYSTEM/OBJECT_TRACKER_SENSOR_FUSION/RADAR_HOMOGENEOUS_FUSION/GATING/MEASUREMENT_TO_TRACK_GATING_AND_LOGLIKELIHOOD_COMPUTATION/GATE_MEASUREMENTS_AND_COMPUTE_LIKELIHOOD ==
  GatedMeasFlagArrayIn : Inport
  Meas : Inport  Port=2
  nMeas : Inport  Port=3
  TrackStateVector : Inport  Port=4
  TrackErrCov : Inport  Port=5
  TrackIdx : Inport  Port=6
  SnsrParam : Inport  Port=7
  LogLikelihoodArrayIn : Inport  Port=8
  For Iterator : ForIterator  ResetStates=reset  IterationSource=external
  GATE_MEASUREMENT_AND_COMPUTE_LOG_LIKELIHOOD : Subsystem
  GET_DATA : Subsystem
  MAHALANOBIS_DISTANCE : Subsystem
  GatedMeasFlagArray : Outport
  LogLikelihoodArray1 : Outport  Port=2
  wires:
  nMeas/1 -> For Iterator/1
  Meas/1 -> GET_DATA/1(MEAS)
  SnsrParam/1 -> GET_DATA/2(SNSR_PARAM)
  GET_DATA/1(measVector) -> MAHALANOBIS_DISTANCE/1(meas)
  TrackStateVector/1 -> MAHALANOBIS_DISTANCE/3(TrackStateVector)
  TrackErrCov/1 -> MAHALANOBIS_DISTANCE/4(TrackErrCov)
  GET_DATA/2(measCov) -> MAHALANOBIS_DISTANCE/2(measCov)
  For Iterator/1 -> GET_DATA/3(measIdx), GATE_MEASUREMENT_AND_COMPUTE_LOG_LIKELIHOOD/7(measIdx)
  MAHALANOBIS_DISTANCE/1(mDist) -> GATE_MEASUREMENT_AND_COMPUTE_LOG_LIKELIHOOD/1(mDist)
  GET_DATA/3(P_D) -> GATE_MEASUREMENT_AND_COMPUTE_LOG_LIKELIHOOD/6(P_D)
  MAHALANOBIS_DISTANCE/2(innovCov) -> GATE_MEASUREMENT_AND_COMPUTE_LOG_LIKELIHOOD/4(innovCov)
  TrackIdx/1 -> GATE_MEASUREMENT_AND_COMPUTE_LOG_LIKELIHOOD/3(TrackIdx)
  GatedMeasFlagArrayIn/1 -> GATE_MEASUREMENT_AND_COMPUTE_LOG_LIKELIHOOD/2(GatedMeasFlagIn)
  LogLikelihoodArrayIn/1 -> GATE_MEASUREMENT_AND_COMPUTE_LOG_LIKELIHOOD/5(LogLikelihoodArrayIn)
  GATE_MEASUREMENT_AND_COMPUTE_LOG_LIKELIHOOD/2(LogLikelihoodArray) -> LogLikelihoodArray1/1
  GATE_MEASUREMENT_AND_COMPUTE_LOG_LIKELIHOOD/1(GatedMeasFlagArray) -> GatedMeasFlagArray/1

== system Fusion_Frame_Model_Architecture/SENSOR_FUSION_SYSTEM/OBJECT_TRACKER_SENSOR_FUSION/RADAR_HOMOGENEOUS_FUSION/GATING/MEASUREMENT_TO_TRACK_GATING_AND_LOGLIKELIHOOD_COMPUTATION/GET_DATA ==
  Meas : Inport
  TrackParamPred : Inport  Port=2
  TrackIdx : Inport  Port=3
  Bus Selector : BusSelector  OutputSignals=StateParam
  Bus Selector1 : BusSelector  OutputSignals=px,vx,ax,py,vy,ay,ErrCOV
  Bus Selector2 : BusSelector  OutputSignals=ValidCumulativeMeasCount
  Mux : Mux  Inputs=6
  Reshape : Reshape  OutputDimensionality=Column vector (2-D)
  Selector : Selector  NumberOfDimensions=2  InputPortWidth=100  IndexOptions=Select all,Index vector (port)  Indices=[1 3],1  OutputSizes=1,1
  Selector1 : Selector  NumberOfDimensions=2  InputPortWidth=3  IndexOptions=Select all,Index vector (port)  Indices=[1 3],1  OutputSizes=1,1
  Width : Width
  nMeas : Outport
  StateVector : Outport  Port=2
  StateErrCov : Outport  Port=3
  wires:
  TrackParamPred/1 -> Selector/1
  TrackIdx/1 -> Selector/2
  Selector/1 -> Bus Selector/1
  Reshape/1 -> StateVector/1
  Bus Selector/1 -> Bus Selector1/1  "<StateParam>"
  Bus Selector1/7 -> StateErrCov/1  "<ErrCOV>"
  Bus Selector1/1 -> Mux/1  "<px>"
  Bus Selector1/2 -> Mux/2  "<vx>"
  Bus Selector1/3 -> Mux/3  "<ax>"
  Bus Selector1/4 -> Mux/4  "<py>"
  Bus Selector1/5 -> Mux/5  "<vy>"
  Bus Selector1/6 -> Mux/6  "<ay>"
  Mux/1 -> Reshape/1
  Meas/1 -> Bus Selector2/1
  Bus Selector2/1 -> Width/1, Selector1/1  "<ValidCumulativeMeasCount>"
  Width/1 -> Selector1/2
  Selector1/1 -> nMeas/1

== system Fusion_Frame_Model_Architecture/SENSOR_FUSION_SYSTEM/OBJECT_TRACKER_SENSOR_FUSION/RADAR_HOMOGENEOUS_FUSION/SIMPLYFIED_DBSCAN_FOR_RADAR_MEASUREMENT_GROUPING/DBSCAN_MEASUREMENT_GROUPING/CHECK_IF_CLUSTER_FORMED ==
  nPts : Inport
  Constant : Constant  Value=uint16(0)
  GreaterThan : RelationalOperator  Operator=>  OutDataTypeStr=boolean  RndMeth=Simplest
  Logical Operator : Logic  Operator=NOT  AllPortsSameDT=off  OutDataTypeStr=boolean
  NoUpd : Outport
  Upd : Outport  Port=2
  wires:
  nPts/1 -> GreaterThan/1
  GreaterThan/1 -> Logical Operator/1, Upd/1
  Constant/1 -> GreaterThan/2
  Logical Operator/1 -> NoUpd/1

== system Fusion_Frame_Model_Architecture/SENSOR_FUSION_SYSTEM/OBJECT_TRACKER_SENSOR_FUSION/RADAR_HOMOGENEOUS_FUSION/SIMPLYFIED_DBSCAN_FOR_RADAR_MEASUREMENT_GROUPING/DBSCAN_MEASUREMENT_GROUPING/COMPUTE_MEAN_IF_CLUSTER_FORMED ==
  CLSTR_DATA : Inport
  meas : Inport  Port=2
  Enable : EnablePort
  COMPUTE_COVARIANCE : Subsystem
  COMPUTE_COVARIANCE_SUM : Subsystem  TreatAsAtomicUnit=on
  COMPUTE_MEAN : Subsystem
  COMPUTE_MEAN_SUM : Subsystem  TreatAsAtomicUnit=on
  GET_DATA : Subsystem
  CLSTR_CNTR_UPD : Outport
  CLSTR_COV_UPD : Outport  Port=2
  wires:
  GET_DATA/1(nPts) -> [nPts], COMPUTE_MEAN_SUM/2(nPoints), COMPUTE_MEAN/2(n), COMPUTE_COVARIANCE_SUM/3(nPoints)
  GET_DATA/2(<ClusterMember>) -> COMPUTE_COVARIANCE_SUM/4(ClusterMembers), [ClstrMembers]
  [Meas] -> COMPUTE_COVARIANCE_SUM/2(MeasArray)
  meas/1 -> [Meas], COMPUTE_MEAN_SUM/3(MeasArray)
  [ClstrMembers] -> COMPUTE_MEAN_SUM/1(ClusterMembers)
  COMPUTE_COVARIANCE/1(Covariance) -> CLSTR_COV_UPD/1
  [nPts] -> COMPUTE_COVARIANCE/2(n)
  COMPUTE_MEAN/1(mean) -> CLSTR_CNTR_UPD/1, COMPUTE_COVARIANCE_SUM/1(mean)
  CLSTR_DATA/1 -> GET_DATA/1(CLSTR)
  COMPUTE_MEAN_SUM/1(ClusterMeanSUM) -> COMPUTE_MEAN/1(mean_sum)
  COMPUTE_COVARIANCE_SUM/1(ClusterCovSUM) -> COMPUTE_COVARIANCE/1(covariance_sum)

== system Fusion_Frame_Model_Architecture/SENSOR_FUSION_SYSTEM/OBJECT_TRACKER_SENSOR_FUSION/RADAR_HOMOGENEOUS_FUSION/SIMPLYFIED_DBSCAN_FOR_RADAR_MEASUREMENT_GROUPING/DBSCAN_MEASUREMENT_GROUPING/FORM_CLUSTER ==
  idx_i : Inport
  measArray : Inport  Port=2
  CLSTR_DATA : Inport  Port=3
  CHECK_CONDITION : Subsystem
  DBSCAN : Subsystem
  If : If  IfExpression=u1 ~= 0
  MERGE_SIGNALS : Subsystem
  NO_CLUSTER_FORMED : Subsystem  TreatAsAtomicUnit=on
  nPts : Outport
  isMeasVisited : Outport  Port=2
  wires:
  idx_i/1 -> DBSCAN/3(idx_i), CHECK_CONDITION/1(idx_i)
  CLSTR_DATA/1 -> CHECK_CONDITION/2(CLSTR_in)
  CHECK_CONDITION/1(isNotVisited) -> If/1
  If/1 -> DBSCAN/Action
  If/2 -> NO_CLUSTER_FORMED/Action
  measArray/1 -> DBSCAN/2(measArray)
  NO_CLUSTER_FORMED/1(CLSTR_DATA_NO_UPD) -> MERGE_SIGNALS/1(CLSTR_NO_UPD)
  NO_CLUSTER_FORMED/2(nPtsEpsNoUpd) -> MERGE_SIGNALS/2(nPtsEpsNoUpd)
  DBSCAN/1(nPtsEps) -> MERGE_SIGNALS/3(nPtsUpd)
  MERGE_SIGNALS/2(CLSTR_DATA) -> isMeasVisited/1
  CHECK_CONDITION/2(CLSTR_out) -> DBSCAN/1(CLSTR_DATA), NO_CLUSTER_FORMED/1(CLSTR_DATA)
  DBSCAN/2(CLSTR_DATA_UPD) -> MERGE_SIGNALS/4(CLSTR_UPD)
  MERGE_SIGNALS/1(nPtsEps) -> nPts/1

== system Fusion_Frame_Model_Architecture/SENSOR_FUSION_SYSTEM/OBJECT_TRACKER_SENSOR_FUSION/RADAR_HOMOGENEOUS_FUSION/SIMPLYFIED_DBSCAN_FOR_RADAR_MEASUREMENT_GROUPING/DBSCAN_MEASUREMENT_GROUPING/IF_CLUSTER_NOT_FORMED ==
  Enable : EnablePort
  Constant : Constant  Value=single(zeros(2,1))  VectorParams1D=off
  Constant1 : Constant  Value=single(zeros(2,2))  VectorParams1D=off
  Mean : Outport
  Cov : Outport  Port=2
  wires:
  Constant/1 -> Mean/1
  Constant1/1 -> Cov/1

== system Fusion_Frame_Model_Architecture/SENSOR_FUSION_SYSTEM/OBJECT_TRACKER_SENSOR_FUSION/RADAR_HOMOGENEOUS_FUSION/SIMPLYFIED_DBSCAN_FOR_RADAR_MEASUREMENT_GROUPING/DBSCAN_MEASUREMENT_GROUPING/MERGE_SIGNALS ==
  MeanNoUpd : Inport
  CovNoUpd : Inport  Port=2
  MeanUpd : Inport  Port=3
  CovUpd : Inport  Port=4
  CLSTR_DATA : Inport  Port=5
  Flag : Inport  Port=6
  GET_DATA_FROM_BUS : Subsystem
  SET_DATA_TO_BUS : Subsystem
  UPDATE_CLUSTER_DATA : Subsystem
  CLSTR_DATA_UPD : Outport
  wires:
  GET_DATA_FROM_BUS/1(<ClusterCenter>) -> UPDATE_CLUSTER_DATA/1(Center_ARRAY)
  GET_DATA_FROM_BUS/2(<ClusterCovariance>) -> UPDATE_CLUSTER_DATA/2(Cov_ARRAY)
  GET_DATA_FROM_BUS/3(<nClusters>) -> UPDATE_CLUSTER_DATA/3(ID)
  UPDATE_CLUSTER_DATA/1(CenterUpd) -> SET_DATA_TO_BUS/2(Mean_ARRAY)
  UPDATE_CLUSTER_DATA/2(CovUpd) -> SET_DATA_TO_BUS/3(Cov_ARRAY)
  MeanUpd/1 -> UPDATE_CLUSTER_DATA/4(mean1)
  MeanNoUpd/1 -> UPDATE_CLUSTER_DATA/5(mean2)
  CovNoUpd/1 -> UPDATE_CLUSTER_DATA/7(Cov2)
  Flag/1 -> UPDATE_CLUSTER_DATA/8(FLAG)
  CovUpd/1 -> UPDATE_CLUSTER_DATA/6(Cov1)
  CLSTR_DATA/1 -> SET_DATA_TO_BUS/1(CLSTR_DATA), GET_DATA_FROM_BUS/1(CLSTR_DATA)
  SET_DATA_TO_BUS/1("CLSTR_DATA_UPD ") -> CLSTR_DATA_UPD/1

== system Fusion_Frame_Model_Architecture/SENSOR_FUSION_SYSTEM/OBJECT_TRACKER_SENSOR_FUSION/RADAR_HOMOGENEOUS_FUSION/STATE_PREDICTION/TRACK_STATE_PREDICTION/GET_DATA ==
  TrackParamPred : Inport
  TrackIdx : Inport  Port=2
  Bus Selector : BusSelector  OutputSignals=StateParam
  Bus Selector1 : BusSelector  OutputSignals=px,vx,ax,py,vy,ay,ErrCOV
  Mux : Mux  Inputs=6
  Reshape : Reshape  OutputDimensionality=Column vector (2-D)
  Selector : Selector  NumberOfDimensions=2  InputPortWidth=100  IndexOptions=Select all,Index vector (port)  Indices=[1 3],1  OutputSizes=1,1
  StateVector : Outport
  StateErrCov : Outport  Port=2
  wires:
  TrackParamPred/1 -> Selector/1
  TrackIdx/1 -> Selector/2
  Selector/1 -> Bus Selector/1
  Reshape/1 -> StateVector/1
  Bus Selector/1 -> Bus Selector1/1  "<StateParam>"
  Bus Selector1/7 -> StateErrCov/1  "<ErrCOV>"
  Bus Selector1/1 -> Mux/1  "<px>"
  Bus Selector1/2 -> Mux/2  "<vx>"
  Bus Selector1/3 -> Mux/3  "<ax>"
  Bus Selector1/4 -> Mux/4  "<py>"
  Bus Selector1/5 -> Mux/5  "<vy>"
  Bus Selector1/6 -> Mux/6  "<ay>"
  Mux/1 -> Reshape/1

== system Fusion_Frame_Model_Architecture/SENSOR_FUSION_SYSTEM/OBJECT_TRACKER_SENSOR_FUSION/RADAR_HOMOGENEOUS_FUSION/STATE_PREDICTION/TRACK_STATE_PREDICTION/SET_DATA ==
  StatePred : Inport
  PredStateErrCov : Inport  Port=2
  objIdx : Inport  Port=3
  StateParamArray : Inport  Port=4
  Assignment1 : Assignment  NumberOfDimensions=2  DiagnosticForDimensions=Warning  IndexOptions=Assign all,Index vector (port)  Indices=1,1  OutputSizes=1,1
  Bus Creator : BusCreator  Inputs=8  OutDataTypeStr=Bus: TrackParamBus  NonVirtualBus=on
      settings: InheritFromInputs=off
  Bus Creator1 : BusCreator  Inputs=7  OutDataTypeStr=Bus: StateParamBus  NonVirtualBus=on
      settings: InheritFromInputs=off
  Bus Selector : BusSelector  OutputSignals=id,StateParam,StateCamSpecificParam,StateRadSpecificParam,StateParamAccuracy,SensorCatch,TrackQuality,TrackStatus
  Selector : Selector  NumberOfDimensions=2  InputPortWidth=3  IndexOptions=Select all,Index vector (port)  Indices=[1 3],1  OutputSizes=1,1
  Selector1 : Selector  InputPortWidth=6  IndexOptions=Index vector (dialog)  Indices=1  OutputSizes=1
  Selector2 : Selector  InputPortWidth=6  IndexOptions=Index vector (dialog)  Indices=2  OutputSizes=1
  Selector3 : Selector  InputPortWidth=6  IndexOptions=Index vector (dialog)  Indices=3  OutputSizes=1
  Selector4 : Selector  InputPortWidth=6  IndexOptions=Index vector (dialog)  Indices=4  OutputSizes=1
  Selector5 : Selector  InputPortWidth=6  IndexOptions=Index vector (dialog)  Indices=5  OutputSizes=1
  Selector6 : Selector  InputPortWidth=6  IndexOptions=Index vector (dialog)  Indices=6  OutputSizes=1
  Terminator : Terminator
  StateParam : Outport
  wires:
  StatePred/1 -> Selector6/1, Selector5/1, Selector4/1, Selector1/1, Selector2/1, Selector3/1
  Selector2/1 -> Bus Creator1/2  "vx"
  Selector4/1 -> Bus Creator1/4  "py"
  Selector3/1 -> Bus Creator1/3  "ax"
  Selector5/1 -> Bus Creator1/5  "vy"
  Selector1/1 -> Bus Creator1/1  "px"
  Selector6/1 -> Bus Creator1/6  "ay"
  Bus Creator1/1 -> [idx]
  PredStateErrCov/1 -> Bus Creator1/7  "ErrCOV"
  Bus Selector/1 -> Bus Creator/1  "<id>"
  Bus Selector/3 -> Bus Creator/3  "<StateCamSpecificParam>"
  Bus Selector/4 -> Bus Creator/4  "<StateRadSpecificParam>"
  Bus Selector/5 -> Bus Creator/5  "<StateParamAccuracy>"
  Bus Selector/6 -> Bus Creator/6  "<SensorCatch>"
  Bus Selector/7 -> Bus Creator/7  "<TrackQuality>"
  Bus Selector/8 -> Bus Creator/8  "<TrackStatus>"
  StateParamArray/1 -> [TrackArray], Selector/1
  objIdx/1 -> [objIdx], Selector/2
  Selector/1 -> Bus Selector/1
  Bus Creator/1 -> Assignment1/2
  Assignment1/1 -> StateParam/1
  [objIdx] -> Assignment1/3
  [TrackArray] -> Assignment1/1
  Bus Selector/2 -> Terminator/1  "<StateParam>"
  [idx] -> Bus Creator/2

== system Fusion_Frame_Model_Architecture/SENSOR_FUSION_SYSTEM/OBJECT_TRACKER_SENSOR_FUSION/RADAR_HOMOGENEOUS_FUSION/STATE_PREDICTION/TRACK_STATE_PREDICTION/StatePredictionLinearModels ==
  StateVectorCA : Inport
  PrevStateErrorCov : Inport  Port=2
  Add : Sum
  Constant : Constant  Value=StateTranMatrix_CA
  Constant1 : Constant  Value=ProcessNoiseCovMat_CA
  Matrix Multiply : Product  Multiplication=Matrix(*)
  Matrix Multiply1 : Product  Inputs=3  Multiplication=Matrix(*)
  Transpose : Math  Operator=transpose  SaturateOnIntegerOverflow=on
  StatePred : Outport
  PriorStateErrorCov : Outport  Port=2
  wires:
  Add/1 -> PriorStateErrorCov/1
  Matrix Multiply/1 -> StatePred/1
  StateVectorCA/1 -> Matrix Multiply/2
  Constant1/1 -> Add/2
  Transpose/1 -> Matrix Multiply1/3
  Matrix Multiply1/1 -> Add/1
  Constant/1 -> Transpose/1, Matrix Multiply1/1, Matrix Multiply/1
  PrevStateErrorCov/1 -> Matrix Multiply1/2

== system Fusion_Frame_Model_Architecture/SENSOR_FUSION_SYSTEM/OBJECT_TRACKER_SENSOR_FUSION/SENSOR_LAYOUT_AND_CHRACTERIZATION/PRE_COMPUTE_SENSOR_FOV_GRID/COMPUTE_CAMERA_SNSR_GRID/ComputeCoverageANDConfidence ==
  RegionConfidenceArray : Inport
  nGridCells : Inport  Port=2
  GridIDVector : Inport  Port=3
  GridParam : Inport  Port=4
  SensorID : Inport  Port=5
  SensorExtrinsic : Inport  Port=6
  SensorIntrinsic : Inport  Port=7
  FOVOverlapArray : Inport  Port=8
  Compute_Cell_X_and_Y_index : Subsystem
  For Iterator : ForIterator  ResetStates=reset  IterationSource=external
  SET_DATA : Subsystem
  RegionConfidence : Outport
  FOVOverlap : Outport  Port=2
  wires:
  nGridCells/1 -> For Iterator/1
  For Iterator/1 -> SET_DATA/1(GridIndex), Compute_Cell_X_and_Y_index/1(CellIndex)
  GridParam/1 -> Compute_Cell_X_and_Y_index/3(GridParam)
  GridIDVector/1 -> Compute_Cell_X_and_Y_index/2(GridID_vec)
  SensorExtrinsic/1 -> Compute_Cell_X_and_Y_index/4(SensorExtrinsicParam)
  SensorIntrinsic/1 -> Compute_Cell_X_and_Y_index/5(SensorIntrinsicParam)
  RegionConfidenceArray/1 -> SET_DATA/2(RegionConfiArray)
  Compute_Cell_X_and_Y_index/1(RegionConfidence) -> SET_DATA/5(confi)
  SensorID/1 -> SET_DATA/4(SnsrIndex)
  FOVOverlapArray/1 -> SET_DATA/3(FOVOverlapArray)
  Compute_Cell_X_and_Y_index/2(FOVOverlap) -> SET_DATA/6(overlap)
  SET_DATA/1(RegionConfidence) -> RegionConfidence/1
  SET_DATA/2(FOVOverlap) -> FOVOverlap/1

== system Fusion_Frame_Model_Architecture/SENSOR_FUSION_SYSTEM/OBJECT_TRACKER_SENSOR_FUSION/SENSOR_LAYOUT_AND_CHRACTERIZATION/PRE_COMPUTE_SENSOR_FOV_GRID/COMPUTE_CAMERA_SNSR_GRID/GET_SENSOR_PARAMETERS ==
  SensorID : Inport
  SensorParam : Inport  Port=2
  Bus Selector : BusSelector  OutputSignals=CameraIntrinsics,CameraExtrinsics
  Bus Selector1 : BusSelector  OutputSignals=CameraType
  Selector : Selector  NumberOfDimensions=2  InputPortWidth=3  IndexOptions=Select all,Index vector (port)  Indices=[1 3],1  OutputSizes=1,1
  Selector1 : Selector  NumberOfDimensions=2  InputPortWidth=3  IndexOptions=Select all,Index vector (port)  Indices=[1 3],1  OutputSizes=1,1
  extrinsic : Outport
  intrinsic : Outport  Port=2
  wires:
  Bus Selector/2 -> Selector/1  "<CameraExtrinsics>"
  Bus Selector1/1 -> Selector1/2  "<CameraType>"
  Selector/1 -> extrinsic/1, Bus Selector1/1
  SensorID/1 -> Selector/2
  SensorParam/1 -> Bus Selector/1
  Bus Selector/1 -> Selector1/1  "<CameraIntrinsics>"
  Selector1/1 -> intrinsic/1

== system Fusion_Frame_Model_Architecture/SENSOR_FUSION_SYSTEM/OBJECT_TRACKER_SENSOR_FUSION/SENSOR_LAYOUT_AND_CHRACTERIZATION/PRE_COMPUTE_SENSOR_FOV_GRID/COMPUTE_RADAR_SNSR_GRID/ComputeCoverageANDConfidence ==
  RegionConfidenceArray : Inport
  nGridCells : Inport  Port=2
  GridIDVector : Inport  Port=3
  GridParam : Inport  Port=4
  SensorID : Inport  Port=5
  SensorExtrinsic : Inport  Port=6
  SensorIntrinsic : Inport  Port=7
  FOVOverlapArray : Inport  Port=8
  Compute_Cell_X_and_Y_index : Subsystem
  For Iterator : ForIterator  ResetStates=reset  IterationSource=external
  SET_DATA : Subsystem
  RegionConfidence : Outport
  FOVOverlap : Outport  Port=2
  wires:
  nGridCells/1 -> For Iterator/1
  For Iterator/1 -> SET_DATA/1(GridIndex), Compute_Cell_X_and_Y_index/1(CellIndex)
  GridParam/1 -> Compute_Cell_X_and_Y_index/3(GridParam)
  GridIDVector/1 -> Compute_Cell_X_and_Y_index/2(GridID_vec)
  SensorExtrinsic/1 -> Compute_Cell_X_and_Y_index/4(SensorExtrinsicParam)
  SensorIntrinsic/1 -> Compute_Cell_X_and_Y_index/5(SensorIntrinsicParam)
  RegionConfidenceArray/1 -> SET_DATA/2(RegionConfiArray)
  Compute_Cell_X_and_Y_index/1(RegionConfidence) -> SET_DATA/5(confi)
  SensorID/1 -> SET_DATA/4(SnsrIndex)
  FOVOverlapArray/1 -> SET_DATA/3(FOVOverlapArray)
  Compute_Cell_X_and_Y_index/2(FOVOverlap) -> SET_DATA/6(overlap)
  SET_DATA/1(RegionConfidence) -> RegionConfidence/1
  SET_DATA/2(FOVOverlap) -> FOVOverlap/1

== system Fusion_Frame_Model_Architecture/SENSOR_FUSION_SYSTEM/OBJECT_TRACKER_SENSOR_FUSION/SENSOR_LAYOUT_AND_CHRACTERIZATION/PRE_COMPUTE_SENSOR_FOV_GRID/COMPUTE_RADAR_SNSR_GRID/GET_SENSOR_PARAMETERS ==
  SensorID : Inport
  SensorParam : Inport  Port=2
  Bus Selector : BusSelector  OutputSignals=RadarIntrinsics,RadarExtrinsics
  Bus Selector1 : BusSelector  OutputSignals=RadarType
  Selector : Selector  NumberOfDimensions=2  InputPortWidth=3  IndexOptions=Select all,Index vector (port)  Indices=[1 3],1  OutputSizes=1,1
  Selector1 : Selector  NumberOfDimensions=2  InputPortWidth=3  IndexOptions=Select all,Index vector (port)  Indices=[1 3],1  OutputSizes=1,1
  extrinsic : Outport
  intrinsic : Outport  Port=2
  wires:
  Bus Selector/2 -> Selector/1  "<RadarExtrinsics>"
  Bus Selector1/1 -> Selector1/2  "<RadarType>"
  Selector/1 -> extrinsic/1, Bus Selector1/1
  SensorID/1 -> Selector/2
  SensorParam/1 -> Bus Selector/1
  Bus Selector/1 -> Selector1/1  "<RadarIntrinsics>"
  Selector1/1 -> intrinsic/1
